simulink model "xboxControl"  (R2021b)
settings: Solver=VariableStepAuto  StartTime=0.0  StopTime=inf  RelTol=1e-3
libraries: vrlib x1
settings Model: Creator=godet  LastModifiedBy=godet

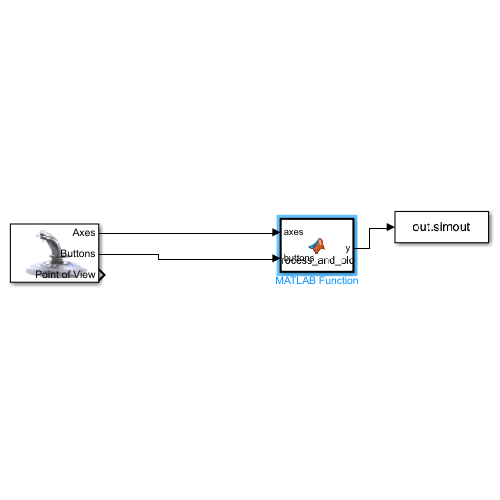
[thumbnail: Simulink's stored preview of the top-level diagram]
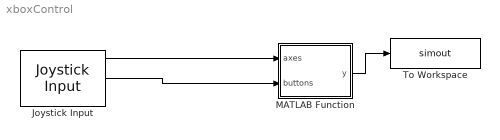
== system xboxControl ==
  Joystick Input : vrlib/Joystick Input  joyid=1  adjustports=on  forcefeed=off
  MATLAB Function : MATLAB Function  TreatAsAtomicUnit=on
  To Workspace : ToWorkspace  VariableName=simout  SaveFormat=Timeseries  SampleTime=-1
      settings: MaxDataPoints=1
  wires:
  Joystick Input/1 -> MATLAB Function/1(axes)
  Joystick Input/2 -> MATLAB Function/2(buttons)
  MATLAB Function/1(y) -> To Workspace/1

== matlab function xboxControl/MATLAB Function ==
  data: axes input; buttons input; y output
function y = process_and_plot(axes, buttons)
%serial com for arduino
% serialObj = serial("COM10","baudRate", 9600)
% configureTerminator(serialObj,"CR/LF");
% flush(serialObj);

% This block processes joystick inputs and visualizes the circles

% Initialize persistent variables
persistent prev_x1 prev_y1 prev_x2 prev_y2 h_fig h_circle1 h_circle2;

% Initialize position variables if empty
if isempty(prev_x1)
    prev_x1 = 0;
    prev_y1 = 0;
    prev_x2 = 0;
    prev_y2 = 0;
end

% Initialize figure and handles if empty
if isempty(h_fig)
    h_fig = figure('Name', 'Xbox Controller Visualization');
end

% Check if figure is valid, if not create new one
if ~ishandle(h_fig)
    h_fig = figure('Name', 'Xbox Controller Visualization');
end

% Set up the figure
figure(h_fig);
set(h_fig, 'Position', [100, 100, 500, 500]);

% Initialize circle handles if empty or invalid
if isempty(h_circle1)  || isempty(h_circle2) 
    clf(h_fig);  % Clear the figure
    hold on;
    h_circle1 = plot(prev_x1, prev_y1, 'o', 'MarkerSize', 20, 'MarkerFaceColor', 'w');
    h_circle2 = plot(prev_x2, prev_y2, 'o', 'MarkerSize', 20, 'MarkerFaceColor', 'w');
    
    % Set up the plot
    xlim([-1.2 1.2]);
    ylim([-1.2 1.2]);
    grid on;
    title('Xbox Controller Circles');
    axis square;
    hold off;
end

% Process joystick inputs
% Get joystick positions (with deadzone)
deadzone = 0.1;
% First joystick
x1_raw = axes(1);  % X-axis of first joystick
y1_raw = axes(2);  % Y-axis of first joystick
% Second joystick
x2_raw = axes(4);  % X-axis of second joystick
y2_raw = axes(5);  % Y-axis of second joystick

% Apply deadzone
x1 = applyDeadzone(x1_raw, deadzone);
y1 = applyDeadzone(y1_raw, deadzone);
x2 = applyDeadzone(x2_raw, deadzone);
y2 = applyDeadzone(y2_raw, deadzone);

% Update positions (scale factor determines speed)
scale = 0.1;
x1 = prev_x1 + x1 * scale;
y1 = prev_y1 - y1 * scale;  % Negative because Y-axis is inverted
x2 = prev_x2 + x2 * scale;
y2 = prev_y2 - y2 * scale;

% Keep circles within bounds (-1 to 1)
x1 = bound(x1);
y1 = bound(y1);
x2 = bound(x2);
y2 = bound(y2);

% Store current positions for next iteration
prev_x1 = x1;
prev_y1 = y1;
prev_x2 = x2;
prev_y2 = y2;

% Process button inputs for colors
% Using buttons 1-4 (A,B,X,Y) for first circle
if buttons(1)  % A button - Green
    color1 = 1;
elseif buttons(2)  % B button - Red
    color1 = 2;
elseif buttons(3)  % X button - Blue
    color1 = 3;
elseif buttons(4)  % Y button - Yellow
    color1 = 4;
else
    color1 = 0;  % Default white
end

% Using buttons 5-8 for second circle
if buttons(5)
    color2 = 1;
elseif buttons(6)
    color2 = 2;
elseif buttons(7)
    color2 = 3;
elseif buttons(8)
    color2 = 4;
else
    color2 = 0;
end

% Update visualization
% Update circle positions
set(h_circle1, 'XData', x1, 'YData', y1);
set(h_circle2, 'XData', x2, 'YData', y2);

% Update colors based on color values
% color1 and color2: 0=white, 1=green, 2=red, 3=blue, 4=yellow
colors = {'w', 'g', 'r', 'b', 'y'};
color_idx1 = color1 + 1; % Add 1 because MATLAB indices start at 1
color_idx2 = color2 + 1;

set(h_circle1, 'MarkerFaceColor', colors{color_idx1});
set(h_circle2, 'MarkerFaceColor', colors{color_idx2});

% Force drawing update
drawnow limitrate;

%write to arduino
y = x1*10;

end

% Helper function to apply deadzone
function out = applyDeadzone(in, deadzone)
    if abs(in) < deadzone
        out = 0;
    else
        out = in;
    end
end

% Helper function to keep values within bounds
function out = bound(in)
    out = min(max(in, -1), 1);
end
